simulink model "kf"  (R2018b)
settings: Solver=FixedStepAuto  StartTime=0.0  StopTime=15  FixedStep=1e-3  RelTol=1e-3
undefined symbols (not defined in the file or in its folder): Discrete, Time
libraries: simulink x2, ctrlSharedLib x1
settings Model: Creator=jasprit  LastModifiedBy=jasprit
settings SFSimCC: SimUseLocalCustomCode=off
settings RTWCC: RTWUseLocalCustomCode=off

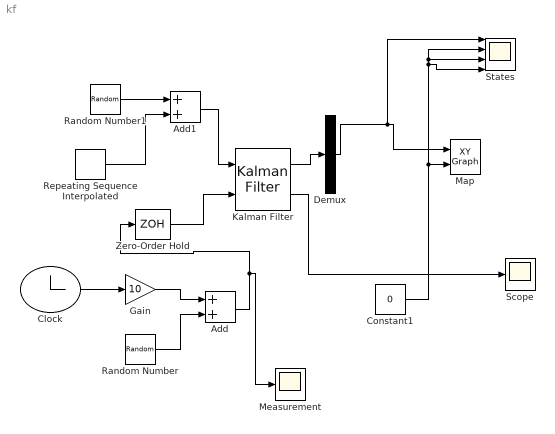
== system kf ==
  Add : Sum
  Add1 : Sum
  Clock : Clock
  Constant1 : Constant  Value=0
  Demux : Demux  Outputs=1
  Gain : Gain  Gain=10
  Kalman Filter : ctrlSharedLib/Kalman Filter  TimeDomain=Discrete-Time  UseCurrentEstimator=on  ModelSource=Individual A, B, C, D matrices  ModelSourceVariable=ss(0.95,1,1,0,1)  A=0  B=1  C=1  D=0  NumberOfStates=1  NumberOfInputs=1  NumberOfOutputs=1  InitialEstimateSource=Dialog  X0=0  P0=10  UseK=off  UseGH=off  NumberOfProcessNoiseInputs=1  G=1  TimeInvariantG=on  H=0  TimeInvariantH=on  Q=0.2  TimeInvariantQ=on  R=0.1  TimeInvariantR=on  N=0  TimeInvariantN=on  AddInputPort=on  AddEnablePort=off  OutputEstimatedY=off  OutputP=on  Ts=-1
      settings: SourceProductBaseCode=CT
  Map : simulink/Sinks/XY Graph  xmin=-1  xmax=1  ymin=-1  ymax=1  st=-1
  "Measurement " : Scope
  Random Number : RandomNumber  Variance=0.1  SampleTime=0.1
  Random Number1 : RandomNumber  Variance=0.8
  Repeating Sequence Interpolated : simulink/Sources/Repeating Sequence Interpolated  OutValues=[30 10 40 20 10].'  TimeValues=[0 3 6 9 12].'  LookUpMeth=Interpolation-Use End Values  tsamp=0.01  OutMin=[]  OutMax=[]  OutDataTypeStr=double  OutputDataTypeScalingMode=double  OutDataType=fixdt(0,8)  OutScaling=2^-10
  Scope : Scope
  States : Scope  NumInputPorts=4
  Zero-Order Hold : ZeroOrderHold  SampleTime=-1
  wires:
  Repeating Sequence Interpolated/1 -> Add1/2
  Kalman Filter/1 -> Demux/1
  Demux/1 -> States/1, Map/1
  Clock/1 -> Gain/1
  Gain/1 -> Add/1
  Random Number/1 -> Add/2
  Add/1 -> Zero-Order Hold/1, "Measurement "/1
  Constant1/1 -> States/4, States/3, States/2, Map/2
  Random Number1/1 -> Add1/1
  Add1/1 -> Kalman Filter/1
  Zero-Order Hold/1 -> Kalman Filter/2
  Kalman Filter/2 -> Scope/1
